simulink model "setup_comp"  (R2023a)
settings: Solver=VariableStepAuto  StartTime=0.0  StopTime=0.5  RelTol=1e-3
settings Model: Creator=isaac  LastModifiedBy=isaac

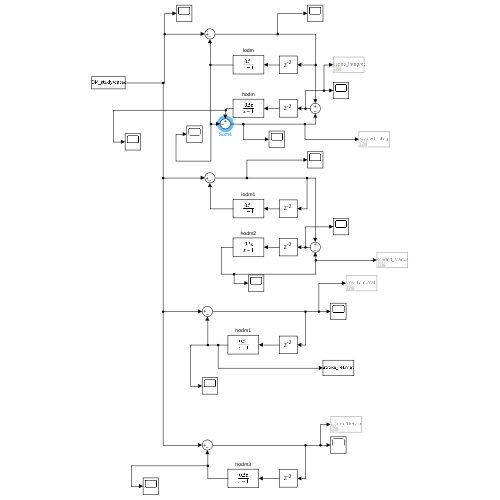
[thumbnail: Simulink's stored preview of the top-level diagram]
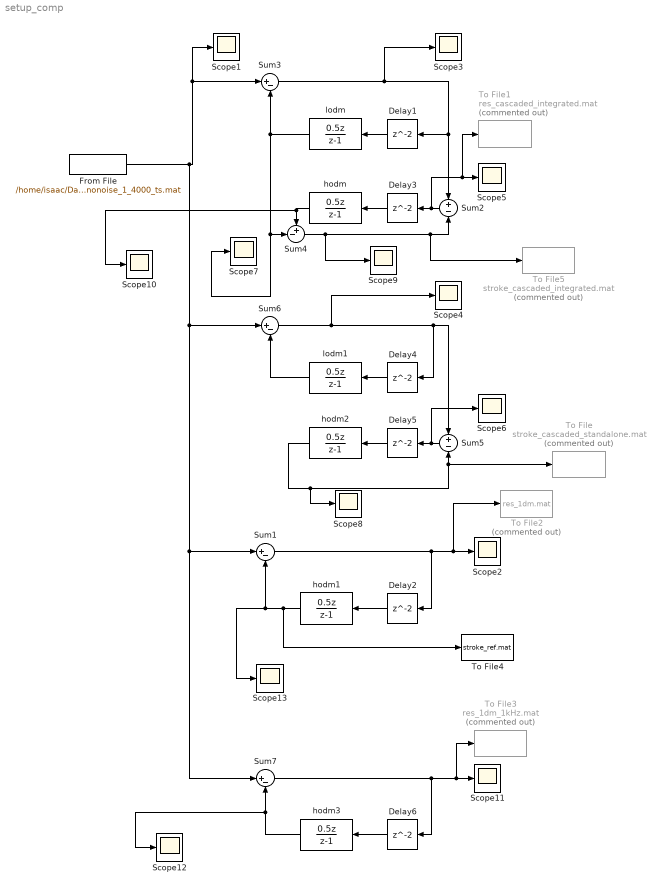
== system setup_comp ==
  Delay{1..5} (5 alike) : Delay  SampleTime=1/4000
  Delay6 : Delay  SampleTime=1/1000
  From File : FromFile  FileName=/home/isaac/Data-Driven-Control-for-AO/2DM_study/data/single_mode_dist_nonoise_1_4000_ts.mat  SampleTime=1/4000
  Scope{1..13} (13 alike) : Scope
  Sum{1,3,6..7} (4 alike) : Sum  Inputs=|+-
  Sum2 : Sum  Inputs=+-
  Sum4 : Sum  Inputs=+-|
  Sum5 : Sum  Inputs=+-
  To File : ToFile  Commented=on  Filename=stroke_cascaded_standalone.mat  MatrixName=data
  To File1 : ToFile  Commented=on  Filename=res_cascaded_integrated.mat  MatrixName=res_cascaded_integrated
  To File2 : ToFile  Commented=on  Filename=res_1dm.mat  MatrixName=res_1dm
  To File3 : ToFile  Commented=on  Filename=res_1dm_1kHz.mat  MatrixName=res_1dm
  To File4 : ToFile  Filename=stroke_ref.mat  MatrixName=data
  To File5 : ToFile  Commented=on  Filename=stroke_cascaded_integrated.mat  MatrixName=data
  hodm : DiscreteTransferFcn  Numerator=[0.5 0]  Denominator=[1 -1]  SampleTime=1/4000
  hodm1 : DiscreteTransferFcn  Numerator=[0.5 0]  Denominator=[1 -1]  SampleTime=1/4000
  hodm2 : DiscreteTransferFcn  Numerator=[0.5 0]  Denominator=[1 -1]  SampleTime=1/4000
  hodm3 : DiscreteTransferFcn  Numerator=[0.5 0]  Denominator=[1 -1]  SampleTime=1/1000
  lodm : DiscreteTransferFcn  Numerator=[0.5 0]  Denominator=[1 -1]  SampleTime=1/1000
  lodm1 : DiscreteTransferFcn  Numerator=[0.5 0]  Denominator=[1 -1]  SampleTime=1/1000
  wires:
  Delay1/1 -> lodm/1
  Sum1/1 -> Scope2/1, To File2/1, Delay2/1
  hodm1/1 -> To File4/1, Scope13/1, Sum1/2
  Delay3/1 -> hodm/1
  Sum3/1 -> Scope3/1, Sum2/1, Delay1/1
  lodm/1 -> Scope7/1, Sum4/2, Sum3/2
  Sum2/1 -> To File1/1, Scope5/1, Delay3/1
  hodm/1 -> Scope10/1, Sum4/1
  Sum4/1 -> Scope9/1, To File5/1, Sum2/2
  Sum5/1 -> Scope6/1, Delay5/1
  Delay4/1 -> lodm1/1
  Sum6/1 -> Sum5/1, Delay4/1, Scope4/1
  lodm1/1 -> Sum6/2
  Delay5/1 -> hodm2/1
  Delay2/1 -> hodm1/1
  hodm3/1 -> Scope12/1, Sum7/2
  From File/1 -> Sum6/1, Sum1/1, Sum7/1, Scope1/1, Sum3/1
  Sum7/1 -> To File3/1, Scope11/1, Delay6/1
  Delay6/1 -> hodm3/1
  hodm2/1 -> Scope8/1, To File/1, Sum5/2
